simulink model "BitConcatDesign"  (R2014a)
settings: Solver=ode45  StartTime=0.0  StopTime=10.0  RelTol=1e-3
libraries: hdlsllib x1
settings Model: Creator=Andrew  LastModifiedBy=Andrew

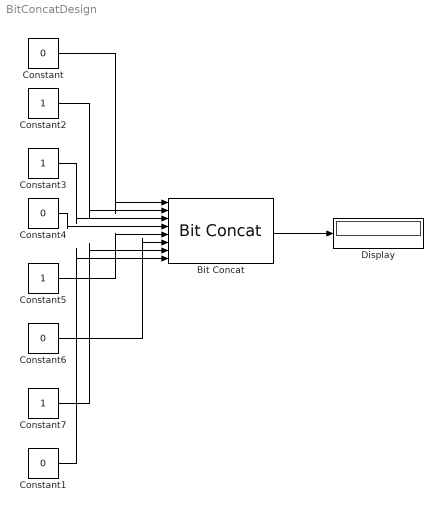
== system BitConcatDesign ==
  Bit Concat : hdlsllib/HDL Operations/Bit Concat  numInputs=8
  Constant{,1,4,6} (4 alike) : Constant  Value=0  OutDataTypeStr=boolean
  Constant{2..3,5,7} (4 alike) : Constant  OutDataTypeStr=boolean
  Display : Display
  wires:
  Constant/1 -> Bit Concat/1
  Constant2/1 -> Bit Concat/2
  Constant3/1 -> Bit Concat/3
  Constant4/1 -> Bit Concat/4
  Constant5/1 -> Bit Concat/5
  Constant6/1 -> Bit Concat/6
  Constant7/1 -> Bit Concat/7
  Constant1/1 -> Bit Concat/8
  Bit Concat/1 -> Display/1
